simulink model "DrawSim"  (R2016b)
settings: Solver=VariableStepAuto  StartTime=0.0  StopTime=1000000  MaxStep=0.1  RelTol=1e-3
undefined symbols (not defined in the file or in its folder): DrawPlane, P
libraries: simulink x10
settings Model: Creator=CFRPG  LastModifiedBy=CFRPG

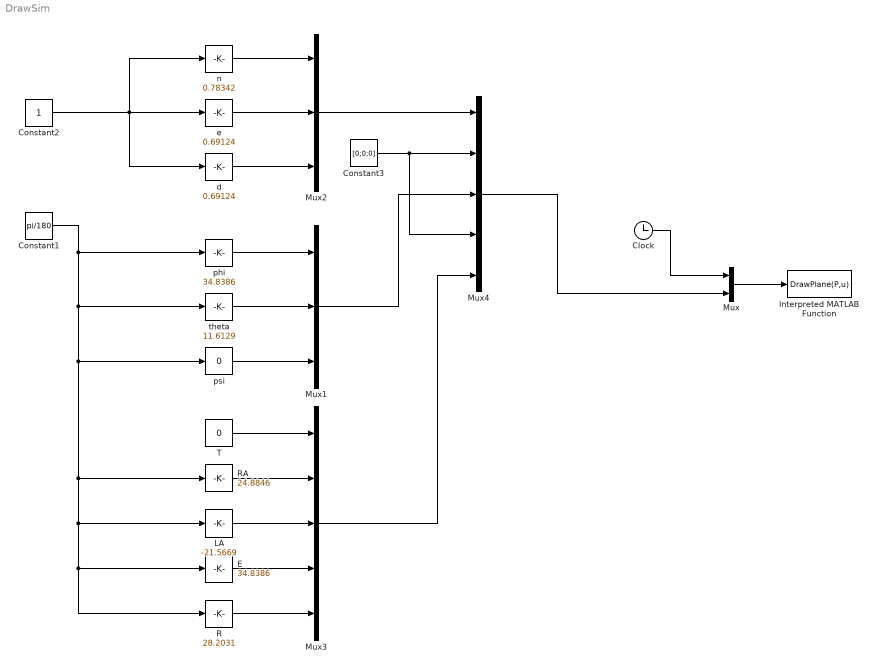
== system DrawSim ==
  Clock : Clock
  Constant1 : Constant  Value=pi/180
  Constant2 : Constant
  Constant3 : Constant  Value=[0;0;0]
  E : simulink/Math Operations/Slider Gain  low=-360  gain=34.8386  high=360
  Interpreted MATLAB Function : MATLABFcn  MATLABFcn=DrawPlane(P,u)  OutputDimensions=0
  LA : simulink/Math Operations/Slider Gain  low=-360  gain=-21.5669  high=360
  Mux : Mux  Inputs=2
  Mux1 : Mux  Inputs=3
  Mux2 : Mux  Inputs=3
  Mux3 : Mux  Inputs=5
  Mux4 : Mux  Inputs=5
  R : simulink/Math Operations/Slider Gain  low=-360  gain=28.2031  high=360
  RA : simulink/Math Operations/Slider Gain  low=-360  gain=24.8846  high=360
  T : Constant  Value=0
  d : simulink/Math Operations/Slider Gain  low=-10  gain=0.69124  high=10
  e : simulink/Math Operations/Slider Gain  low=-10  gain=0.69124  high=10
  n : simulink/Math Operations/Slider Gain  low=-10  gain=0.78342  high=10
  phi : simulink/Math Operations/Slider Gain  low=-360  gain=34.8386  high=360
  psi : simulink/Math Operations/Slider Gain  low=-360  gain=0  high=360
  theta : simulink/Math Operations/Slider Gain  low=-360  gain=11.6129  high=360
  wires:
  Clock/1 -> Mux/1
  Mux/1 -> Interpreted MATLAB Function/1
  Constant1/1 -> R/1, E/1, LA/1, RA/1, psi/1, theta/1, phi/1
  phi/1 -> Mux1/1
  theta/1 -> Mux1/2
  psi/1 -> Mux1/3
  e/1 -> Mux2/2
  n/1 -> Mux2/1
  d/1 -> Mux2/3
  Constant2/1 -> e/1, n/1, d/1
  R/1 -> Mux3/5
  E/1 -> Mux3/4
  LA/1 -> Mux3/3
  RA/1 -> Mux3/2
  T/1 -> Mux3/1
  Mux2/1 -> Mux4/1
  Constant3/1 -> Mux4/4, Mux4/2
  Mux1/1 -> Mux4/3
  Mux3/1 -> Mux4/5
  Mux4/1 -> Mux/2
